simulink model "IEEE_9bus_new_o"  (R2024a)
settings: Solver=ode45  StartTime=0.0  StopTime=10.0  RelTol=1e-3  EnableMultiTasking=on
libraries: spsThreePhaseVIMeasurementLib x21, spsFrequencyPhasorLib x9, spsLoadFlowBusLib x9, spsPower3phInstantaneousLib x9, spsThreePhasePISectionLineLib x6, jailib x3, spsThreePhaseSourceLib x3, spsThreePhaseTransformerTwoWindingsLib x3, sps_lib x1
settings Model: Creator=jp536285  LastModifiedBy=Vaibhav Chaudhary
settings SolverCC: AlgebraicLoopSolver=TrustRegion
settings DataIOCC: LimitDataPoints=on  SaveFormat=Array  ReturnWorkspaceOutputs=off
settings OptimizationCC: LifeSpan=inf
settings DebuggingCC: UnderspecifiedInitializationDetection=Classic  MergeDetectMultiDrivingBlocksExec=none  SolverPrmCheckMsg=warning  StateNameClashWarn=warning  SFUnexpectedBacktrackingDiag=warning  SFNoUnconditionalDefaultTransitionDiag=warning  SFExecutionAtInitializationDiag=none  ArithmeticOperatorsInVariantConditions=warning
settings HardwareCC: ProdBitPerPointer=32  ProdBitPerSizeT=32  ProdBitPerPtrDiffT=32  ProdLargestAtomicFloat=None  ProdIntDivRoundTo=Undefined  ProdEndianess=Unspecified  ProdWordSize=32  ProdHWDeviceType=32-bit Generic
settings ModelReferenceCC: PropagateSignalLabelsOutOfModel=off
settings SFSimCC: SimUseLocalCustomCode=off  CustomCodeUndefinedFunction=UseInterfaceOnly
settings RTWCC: RTWUseLocalCustomCode=off  GPUComputeCapability=3.5
settings CodeAppCC: StateflowObjectComments=on
settings GRTTargetCC: TargetLangStandard=C89/C90 (ANSI)
settings ConfigComp: CovMetricSettings=dw  CovSaveCumulativeToWorkspaceVar=on  CovSaveSingleToWorkspaceVar=on  CovExternalEMLEnable=off
settings SimscapeCC: SimscapeNormalizeSystem=off

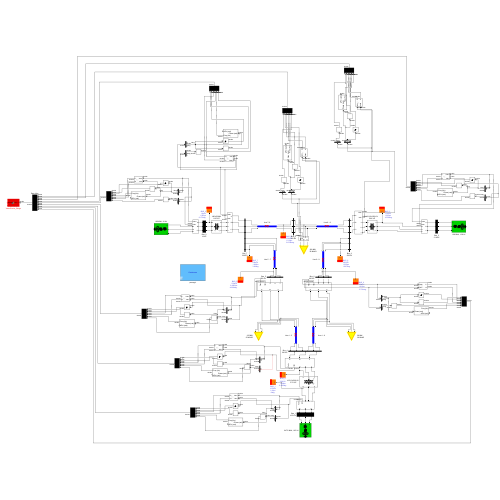
[thumbnail: Simulink's stored preview of the top-level diagram]
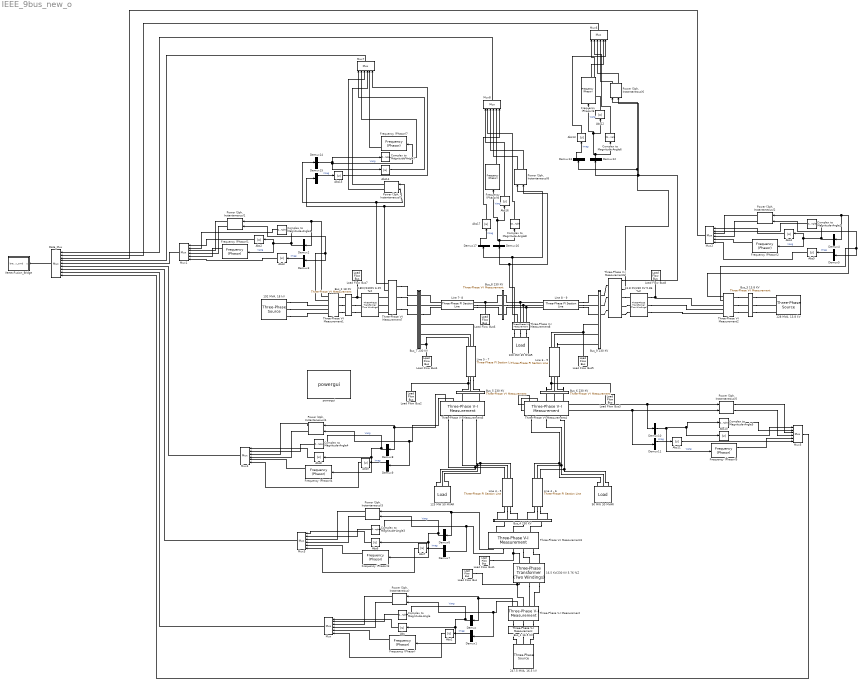
== system IEEE_9bus_new_o ==
  " Line 4 - 6" : spsThreePhasePISectionLineLib/Three-Phase PI Section Line  LConnTagsString=a|b|c  RConnTagsString=A|B|C  Length=100  Frequency=50  Resistances=[ 0.08993 0.224825]  Inductances="[ 1.29e-3  3.22e-3]"  Capacitances=[7.922e-9 4.74e-9]  mask(Three-Phase PI Section Line){}
      mask Display:
      | % This is a new mask on top of the base mask.
      | % Use "View base mask" link below to see the base mask.
      | patch([0.0 0.0 1 1 0.0 0.0 ],[0.4 0.7 0.7 0.4 0.4 0.7],[0 0 1]);
      | patch([0.4 0.4 0.42 0.42],[0.4 0.75 0.75 0.4],[1 0 0]);
      | patch([0.38 0.38 0.57 0.57],[0.7 0.75 0.75 0.7],[1 0 0]);
      | patch([0.53 0.53 0.55 0.55],[0.4 0.75 0.75 0.4],[1 0 0]);
  " Line 6 - 9" : spsThreePhasePISectionLineLib/Three-Phase PI Section Line  LConnTagsString=a|b|c  RConnTagsString=A|B|C  Length=100  Frequency=60  Resistances=[ 0.20631 0.5157]  Inductances="[ 2.38e-3  6.09e-3]"  Capacitances=[17.95e-9 10.55e-9]  mask(Three-Phase PI Section Line){}
      mask Display:
      | % This is a new mask on top of the base mask.
      | % Use "View base mask" link below to see the base mask.
      | patch([0.0 0.0 1 1 0.0 0.0 ],[0.4 0.7 0.7 0.4 0.4 0.7],[0 0 1]);
      | patch([0.4 0.4 0.42 0.42],[0.4 0.75 0.75 0.4],[1 0 0]);
      | patch([0.38 0.38 0.57 0.57],[0.7 0.75 0.75 0.7],[1 0 0]);
      | patch([0.53 0.53 0.55 0.55],[0.4 0.75 0.75 0.4],[1 0 0]);
  100 MW 35 MVAR : jailib/Load  SystemSampleTime=-1  VariantActivationTime=update diagram  AllowFlexibleInterface=on  Latency=0  AutoFrameSizeCalculation=off
      link override Three-Phase Parallel RLC Load: NominalVoltage=230000  ActivePower=100e6  InductivePower=35e6
      settings: SourceProductName=Power Library
  125 MW 50 MVAR : jailib/Load  SystemSampleTime=-1  VariantActivationTime=update diagram  AllowFlexibleInterface=on  Latency=0  AutoFrameSizeCalculation=off
      link override Three-Phase Parallel RLC Load: NominalVoltage=230000  ActivePower=125e6  InductivePower=50e6
      settings: SourceProductName=Power Library
  "128 MVA, 13.8 kV" : spsThreePhaseSourceLib/Three-Phase Source  InternalConnection=Yg  VoltagePhases=off  Voltage=13800  PhaseAngle=0  Voltage_phases=[25e3 25e3 25e3]/sqrt(3)  PhaseAngles_phases=[0 -120 +120]  Frequency=60  NonIdealSource=on  SpecifyImpedance=on  Resistance=0.529  Inductance=0.0140  ShortCircuitLevel=128e6  BaseVoltage=13.8e3  XRratio=100000  BusType=PV  Pref=85000000  Qref=0  Prefabc=[10e3, 10e3, 10e3]  Qrefabc=[0, 0, 0]  Qmin=-inf  Qmax=inf
  13.8 KV/230 KV 5.86 %Z : spsThreePhaseTransformerTwoWindingsLib/Three-Phase Transformer (Two Windings)  Winding1Connection=Yg  Winding2Connection=Yg  CoreType=Three single-phase transformers  SetSaturation=off  Hysteresis=off  DataFile='hysteresis'  SetInitialFlux=off  Measurements=None  UNITS=pu  NominalPower=[ 100e6 , 60 ]  Winding1=[ 13.8e3 , 1e-6 , 0 ]  Winding2=[ 230e3 , 1e-6, 0.0586 ]  Rm=500  Lm=500  L0=0.5  Saturation=[ 0,0 ; 0.0024,1.2 ; 1.0,1.52 ]  InitialFluxes=[ 0.8 , -0.8 , 0.7 ]  BreakLoop=off  DiscreteSolver=Trapezoidal iterative  DataType=off  TransfoNumber=1
  "16.5 KV/230 KV 5.76 %Z     " : spsThreePhaseTransformerTwoWindingsLib/Three-Phase Transformer (Two Windings)  Winding1Connection=Yg  Winding2Connection=Yg  CoreType=Three single-phase transformers  SetSaturation=off  Hysteresis=off  DataFile='hysteresis'  SetInitialFlux=off  Measurements=None  UNITS=pu  NominalPower=[ 100e6 , 60 ]  Winding1=[ 16.5e3 , 1e-6, 0 ]  Winding2=[ 230e3 ,1e-6, 0.0576 ]  Rm=500  Lm=500  L0=0.5  Saturation=[ 0,0 ; 0.0024,1.2 ; 1.0,1.52 ]  InitialFluxes=[ 0.8 , -0.8 , 0.7 ]  BreakLoop=off  DiscreteSolver=Trapezoidal iterative  DataType=off  TransfoNumber=1
  18KV/230KV 6.25 %Z : spsThreePhaseTransformerTwoWindingsLib/Three-Phase Transformer (Two Windings)  Winding1Connection=Yg  Winding2Connection=Yg  CoreType=Three single-phase transformers  SetSaturation=off  Hysteresis=off  DataFile='hysteresis'  SetInitialFlux=off  Measurements=None  UNITS=pu  NominalPower=[ 100e6 , 60 ]  Winding1=[ 18e3 , 1e-6 , 0]  Winding2=[ 230e3 , 1e-6, 0.0625 ]  Rm=500  Lm=500  L0=0.5  Saturation=[ 0,0 ; 0.0024,1.2 ; 1.0,1.52 ]  InitialFluxes=[ 0.8 , -0.8 , 0.7 ]  BreakLoop=off  DiscreteSolver=Trapezoidal iterative  DataType=off  TransfoNumber=1
  "192 MVA, 18 kV" : spsThreePhaseSourceLib/Three-Phase Source  InternalConnection=Yg  VoltagePhases=off  Voltage=18000  PhaseAngle=0  Voltage_phases=[25e3 25e3 25e3]/sqrt(3)  PhaseAngles_phases=[0 -120 +120]  Frequency=60  NonIdealSource=on  SpecifyImpedance=on  Resistance=0.529  Inductance=0.0140  ShortCircuitLevel=192e6  BaseVoltage=18e3  XRratio=100000  BusType=PV  Pref=163000000  Qref=0  Prefabc=[10e3, 10e3, 10e3]  Qrefabc=[0, 0, 0]  Qmin=-inf  Qmax=inf
  "247.5 MVA, 16.5 kV" : spsThreePhaseSourceLib/Three-Phase Source  InternalConnection=Yg  VoltagePhases=off  Voltage=16500  PhaseAngle=0  Voltage_phases=[25e3 25e3 25e3]/sqrt(3)  PhaseAngles_phases=[0 -120 +120]  Frequency=60  NonIdealSource=on  SpecifyImpedance=on  Resistance=0.529  Inductance=0.0140  ShortCircuitLevel=247.5e6  BaseVoltage=16.5e3  XRratio=100000  BusType=swing  Pref=0  Qref=0  Prefabc=[10e3, 10e3, 10e3]  Qrefabc=[0, 0, 0]  Qmin=-Inf  Qmax=Inf
  90 MW 30 MVAR : jailib/Load  SystemSampleTime=-1  VariantActivationTime=update diagram  AllowFlexibleInterface=on  Latency=0  AutoFrameSizeCalculation=off
      link override Three-Phase Parallel RLC Load: NominalVoltage=230000  ActivePower=90e6  InductivePower=30e6
      settings: SourceProductName=Power Library
  Abs{,1..17} (18 alike) : Abs  OutMin=3  OutMax=3  SaturateOnIntegerOverflow=off
  Bus_1 16.5 KV : spsThreePhaseVIMeasurementLib/Three-Phase V-I Measurement  VoltageMeasurement=phase-to-ground  SetLabelV=on  LabelV=Vabc_1  Vpu=on  VpuLL=off  CurrentMeasurement=yes  SetLabelI=on  LabelI=Iabc_1  Ipu=on  Pbase=100e6  Vbase=16.5e3  OutputType=Complex  PhasorSimulation=off  PSBequivalent=0
  Bus_2 18 KV : spsThreePhaseVIMeasurementLib/Three-Phase V-I Measurement  VoltageMeasurement=phase-to-ground  SetLabelV=on  LabelV=Vabc_2  Vpu=on  VpuLL=off  CurrentMeasurement=yes  SetLabelI=on  LabelI=Iabc_2  Ipu=on  Pbase=100e6  Vbase=18e3  OutputType=Complex  PhasorSimulation=off  PSBequivalent=0
  Bus_3 13.8 KV : spsThreePhaseVIMeasurementLib/Three-Phase V-I Measurement  VoltageMeasurement=phase-to-ground  SetLabelV=on  LabelV=Vabc_3  Vpu=on  VpuLL=off  CurrentMeasurement=yes  SetLabelI=on  LabelI=Iabc_3  Ipu=on  Pbase=100e6  Vbase=13.8e3  OutputType=Complex  PhasorSimulation=off  PSBequivalent=0
  Bus_4 230 KV : Subsystem
  Bus_5 230 KV : spsThreePhaseVIMeasurementLib/Three-Phase V-I Measurement  VoltageMeasurement=phase-to-ground  SetLabelV=on  LabelV=Vabc_5  Vpu=on  VpuLL=off  CurrentMeasurement=yes  SetLabelI=on  LabelI=Iabc_5  Ipu=on  Pbase=100e6  Vbase=230e3  OutputType=Complex  PhasorSimulation=off  PSBequivalent=0
  Bus_6 230 KV : spsThreePhaseVIMeasurementLib/Three-Phase V-I Measurement  VoltageMeasurement=phase-to-ground  SetLabelV=on  LabelV=Vabc_6  Vpu=on  VpuLL=off  CurrentMeasurement=yes  SetLabelI=on  LabelI=Iabc_6  Ipu=on  Pbase=100e6  Vbase=230e3  OutputType=Complex  PhasorSimulation=off  PSBequivalent=0
  Bus_7 230 KV : Subsystem
  Bus_8 230 KV : spsThreePhaseVIMeasurementLib/Three-Phase V-I Measurement  VoltageMeasurement=phase-to-ground  SetLabelV=on  LabelV=Vabc_8  Vpu=on  VpuLL=off  CurrentMeasurement=yes  SetLabelI=on  LabelI=Iabc_8  Ipu=on  Pbase=100e6  Vbase=230e3  OutputType=Complex  PhasorSimulation=off  PSBequivalent=0
  Bus_9 230 KV : Subsystem
  Complex to Magnitude-Angle{,1..8} (9 alike) : ComplexToMagnitudeAngle  Output=Angle
  Data_Mux : Mux  Inputs=9
  Demux{,1..17} (18 alike) : Demux  Outputs=3
  Frequency (Phasor){,1..8} (9 alike) : spsFrequencyPhasorLib/Frequency (Phasor)  Fn=60  T=0.1
      settings: LibrarySourceBlock=|
      | sps_lib/Sensors and Measurements/Frequency
      | (Phasor)
  "Line 4 - 5 " : spsThreePhasePISectionLineLib/Three-Phase PI Section Line  LConnTagsString=a|b|c  RConnTagsString=A|B|C  Length=100  Frequency=60  Resistances=[ 0.0529 0.13225]  Inductances="[ 1.192e-3  2.38e-3]"  Capacitances=[8.82e-9 5.188e-9]  mask(Three-Phase PI Section Line){}
      mask Display:
      | % This is a new mask on top of the base mask.
      | % Use "View base mask" link below to see the base mask.
      | patch([0.0 0.0 1 1 0.0 0.0 ],[0.4 0.7 0.7 0.4 0.4 0.7],[0 0 1]);
      | patch([0.4 0.4 0.42 0.42],[0.4 0.75 0.75 0.4],[1 0 0]);
      | patch([0.38 0.38 0.57 0.57],[0.7 0.75 0.75 0.7],[1 0 0]);
      | patch([0.53 0.53 0.55 0.55],[0.4 0.75 0.75 0.4],[1 0 0]);
  "Line 5 - 7 " : spsThreePhasePISectionLineLib/Three-Phase PI Section Line  LConnTagsString=a|b|c  RConnTagsString=A|B|C  Length=100  Frequency=60  Resistances=[ 0.16928 0.4232]  Inductances="[ 2.259e-3  5.64e-3]"  Capacitances=[15.34e-9 9.025e-9]  mask(Three-Phase PI Section Line){}
      mask Display:
      | % This is a new mask on top of the base mask.
      | % Use "View base mask" link below to see the base mask.
      | patch([0.0 0.0 1 1 0.0 0.0 ],[0.4 0.7 0.7 0.4 0.4 0.7],[0 0 1]);
      | patch([0.4 0.4 0.42 0.42],[0.4 0.75 0.75 0.4],[1 0 0]);
      | patch([0.38 0.38 0.57 0.57],[0.7 0.75 0.75 0.7],[1 0 0]);
      | patch([0.53 0.53 0.55 0.55],[0.4 0.75 0.75 0.4],[1 0 0]);
  Line 7- 8 : spsThreePhasePISectionLineLib/Three-Phase PI Section Line  LConnTagsString=a|b|c  RConnTagsString=A|B|C  Length=100  Frequency=60  Resistances=[0.044965 0.11241]  Inductances="[ 1.01e-3  2.02e-3]"  Capacitances=[7.471e-9 4.394e-9]  mask(Three-Phase PI Section Line){}
      mask Display:
      | % This is a new mask on top of the base mask.
      | % Use "View base mask" link below to see the base mask.
      | patch([0.0 0.0 1 1 0.0 0.0 ],[0.4 0.7 0.7 0.4 0.4 0.7],[0 0 1]);
      | patch([0.4 0.4 0.42 0.42],[0.4 0.75 0.75 0.4],[1 0 0]);
      | patch([0.38 0.38 0.57 0.57],[0.7 0.75 0.75 0.7],[1 0 0]);
      | patch([0.53 0.53 0.55 0.55],[0.4 0.75 0.75 0.4],[1 0 0]);
  Line 8 - 9 : spsThreePhasePISectionLineLib/Three-Phase PI Section Line  LConnTagsString=a|b|c  RConnTagsString=A|B|C  Length=100  Frequency=60  Resistances=[ 0.062951 0.15737]  Inductances="[ 1.414e-3  3.53e-3]"  Capacitances=[10.47e-9 6.15e-9]  mask(Three-Phase PI Section Line){}
      mask Display:
      | % This is a new mask on top of the base mask.
      | % Use "View base mask" link below to see the base mask.
      | patch([0.0 0.0 1 1 0.0 0.0 ],[0.4 0.7 0.7 0.4 0.4 0.7],[0 0 1]);
      | patch([0.4 0.4 0.42 0.42],[0.4 0.75 0.75 0.4],[1 0 0]);
      | patch([0.38 0.38 0.57 0.57],[0.7 0.75 0.75 0.7],[1 0 0]);
      | patch([0.53 0.53 0.55 0.55],[0.4 0.75 0.75 0.4],[1 0 0]);
  Load Flow Bus : spsLoadFlowBusLib/Load Flow Bus  LConnTagsString=a  Phases=single  Connectors=on one side  ID=BUS_1  Vbase=16.5e3  Vref=1.04  Vangle=0  VLF=1.04  VLFb=1  VLFc=1  angleLF=0  angleLFb=0  angleLFc=0
      settings: AttributesFormatString=%<ID>\n%<Vbase>V\n%<VLF>pu\n%<angleLF>deg.
  Load Flow Bus1 : spsLoadFlowBusLib/Load Flow Bus  LConnTagsString=a  Phases=single  Connectors=on one side  ID=BUS_4  Vbase=230e3  Vref=1  Vangle=0  VLF=1.026  VLFb=1  VLFc=1  angleLF=-2.226  angleLFb=0  angleLFc=0
      settings: AttributesFormatString=%<ID>\n%<Vbase>V\n%<VLF>pu\n%<angleLF>deg.
  Load Flow Bus2 : spsLoadFlowBusLib/Load Flow Bus  LConnTagsString=a  Phases=single  Connectors=on one side  ID=BUS_5  Vbase=230e3  Vref=1  Vangle=0  VLF=0.9962  VLFb=1  VLFc=1  angleLF=-4.002  angleLFb=0  angleLFc=0
      settings: AttributesFormatString=%<ID>\n%<Vbase>V\n%<VLF>pu\n%<angleLF>deg.
  Load Flow Bus3 : spsLoadFlowBusLib/Load Flow Bus  LConnTagsString=a  Phases=single  Connectors=on one side  ID=BUS_6  Vbase=230e3  Vref=1  Vangle=0  VLF=1.013  VLFb=1  VLFc=1  angleLF=-3.701  angleLFb=0  angleLFc=0
      settings: AttributesFormatString=%<ID>\n%<Vbase>V\n%<VLF>pu\n%<angleLF>deg.
  Load Flow Bus4 : spsLoadFlowBusLib/Load Flow Bus  LConnTagsString=a  Phases=single  Connectors=on one side  ID=BUS_7  Vbase=230e3  Vref=1  Vangle=0  VLF=1.026  VLFb=1  VLFc=1  angleLF=3.62  angleLFb=0  angleLFc=0
      settings: AttributesFormatString=%<ID>\n%<Vbase>V\n%<VLF>pu\n%<angleLF>deg.
  Load Flow Bus5 : spsLoadFlowBusLib/Load Flow Bus  LConnTagsString=a  Phases=single  Connectors=on one side  ID=BUS_9  Vbase=230e3  Vref=1  Vangle=0  VLF=1.032  VLFb=1  VLFc=1  angleLF=1.867  angleLFb=0  angleLFc=0
      settings: AttributesFormatString=%<ID>\n%<Vbase>V\n%<VLF>pu\n%<angleLF>deg.
  Load Flow Bus6 : spsLoadFlowBusLib/Load Flow Bus  LConnTagsString=a  Phases=single  Connectors=on one side  ID=BUS_8  Vbase=230e3  Vref=1  Vangle=0  VLF=1.016  VLFb=1  VLFc=1  angleLF=0.6336  angleLFb=0  angleLFc=0
      settings: AttributesFormatString=%<ID>\n%<Vbase>V\n%<VLF>pu\n%<angleLF>deg.
  Load Flow Bus7 : spsLoadFlowBusLib/Load Flow Bus  LConnTagsString=a  Phases=single  Connectors=on one side  ID=BUS_2  Vbase=18e3  Vref=1.025  Vangle=0  VLF=1.025  VLFb=1  VLFc=1  angleLF=9.173  angleLFb=0  angleLFc=0
      settings: AttributesFormatString=%<ID>\n%<Vbase>V\n%<VLF>pu\n%<angleLF>deg.
  Load Flow Bus8 : spsLoadFlowBusLib/Load Flow Bus  LConnTagsString=a  Phases=single  Connectors=on one side  ID=BUS_3  Vbase=13.8e3  Vref=1.025  Vangle=0  VLF=1.025  VLFb=1  VLFc=1  angleLF=4.558  angleLFb=0  angleLFc=0
      settings: AttributesFormatString=%<ID>\n%<Vbase>V\n%<VLF>pu\n%<angleLF>deg.
  Mux{,1..8} (9 alike) : Mux  Inputs=6
  Power (3ph, Instantaneous){,1..8} (9 alike) : spsPower3phInstantaneousLib/Power (3ph, Instantaneous)
  Three-Phase V-I Measurement{,1..8} (9 alike) : spsThreePhaseVIMeasurementLib/Three-Phase V-I Measurement  VoltageMeasurement=phase-to-ground  SetLabelV=off  LabelV=Vabc  Vpu=on  VpuLL=off  CurrentMeasurement=yes  SetLabelI=off  LabelI=Iabc  Ipu=on  Pbase=100e6  Vbase=500e3  OutputType=Complex  PhasorSimulation=off  PSBequivalent=0
  VertexFusion_Bridge : MATLAB Function  TreatAsAtomicUnit=on
  powergui : sps_lib/powergui  Priority=1  SimulationMode=Continuous  SampleTime=50e-6  frequency=60  Iterations=50  frequencyindice=60  Pbase=10e7  ErrMax=1e-05  UnitsV=kV  UnitsW=MW  buscounter=0  FunctionMessages=off  echomessages=off  EnableUseOfTLC=off  CurrentSourceSwitches=on  DisableSnubberDevices=off  DisableRonSwitches=off  DisableVfSwitches=off  DisplayEquations=off  AutomaticDiscreteSolvers=off  SolverType=Tustin  Interpol=off  ExternalGateDelay=off  methode=off  Ts=0  x0status=blocks  SPID=off  SwTol=0  HookPort=off  NonlinearTolerance=1e-4  nMaxIteration=100  ContinueOnMaxIteration=off  RestoreLinks=warning  ResistiveCurrentMeasurement=off  Frange=[0:2:500]  Ylog=off  Xlog=on  ShowGrid=off  save=off  variable=ZData  structure=0  ZoomFFT=off  StartTime=0.0  cycles=1  DisplayStyle=1  fundamental=60  FreqAxis=off  MaxFrequency=1000  frequencyindicesteady=1  RmsSteady=1  display=off
  wires:
  Three-Phase V-I Measurement/2 -> "Power (3ph, Instantaneous)"/2, Demux1/1
  Demux1/1 -> Abs1/1  "Imag"
  Demux/2 -> Abs/1, Frequency (Phasor)/1, Complex to Magnitude-Angle/1  "Vang"
  Three-Phase V-I Measurement/1 -> "Power (3ph, Instantaneous)"/1, Demux/1
  Abs/1 -> Mux/1
  Complex to Magnitude-Angle/1 -> Mux/2
  "Power (3ph, Instantaneous)"/1 -> Mux/3
  "Power (3ph, Instantaneous)"/2 -> Mux/4
  Frequency (Phasor)/1 -> Mux/5
  Abs1/1 -> Mux/6
  Demux2/2 -> Abs2/1, Frequency (Phasor)1/1, Complex to Magnitude-Angle1/1  "Vang"
  Frequency (Phasor)1/1 -> Mux1/5
  Abs2/1 -> Mux1/1
  Complex to Magnitude-Angle1/1 -> Mux1/2
  Abs3/1 -> Mux1/6
  Demux3/1 -> Abs3/1  "Imag"
  "Power (3ph, Instantaneous)1"/2 -> Mux1/4
  "Power (3ph, Instantaneous)1"/1 -> Mux1/3
  Three-Phase V-I Measurement1/2 -> "Power (3ph, Instantaneous)1"/2, Demux3/1
  Three-Phase V-I Measurement1/1 -> Demux2/1, "Power (3ph, Instantaneous)1"/1
  Three-Phase V-I Measurement2/2 -> "Power (3ph, Instantaneous)2"/2, Demux5/1
  Three-Phase V-I Measurement2/1 -> Demux4/1, "Power (3ph, Instantaneous)2"/1
  "Power (3ph, Instantaneous)2"/1 -> Mux2/3
  "Power (3ph, Instantaneous)2"/2 -> Mux2/4
  Abs5/1 -> Mux2/6
  Abs4/1 -> Mux2/1
  Complex to Magnitude-Angle2/1 -> Mux2/2
  Frequency (Phasor)2/1 -> Mux2/5
  Demux5/1 -> Abs5/1  "Imag"
  Demux4/2 -> Abs4/1, Frequency (Phasor)2/1, Complex to Magnitude-Angle2/1  "Vang"
  Demux6/2 -> Abs6/1, Frequency (Phasor)3/1, Complex to Magnitude-Angle3/1  "Vang"
  Frequency (Phasor)3/1 -> Mux3/5
  Abs6/1 -> Mux3/1
  Complex to Magnitude-Angle3/1 -> Mux3/2
  Abs7/1 -> Mux3/6
  Demux7/1 -> Abs7/1  "Imag"
  "Power (3ph, Instantaneous)3"/2 -> Mux3/4
  "Power (3ph, Instantaneous)3"/1 -> Mux3/3
  Three-Phase V-I Measurement3/2 -> "Power (3ph, Instantaneous)3"/2
  Three-Phase V-I Measurement3/1 -> "Power (3ph, Instantaneous)3"/1, Demux6/1
  Demux8/2 -> Abs8/1, Frequency (Phasor)4/1, Complex to Magnitude-Angle4/1  "Vang"
  Frequency (Phasor)4/1 -> Mux4/5
  Abs8/1 -> Mux4/1
  Complex to Magnitude-Angle4/1 -> Mux4/2
  Abs9/1 -> Mux4/6
  Demux9/1 -> Abs9/1  "Imag"
  "Power (3ph, Instantaneous)4"/2 -> Mux4/4
  "Power (3ph, Instantaneous)4"/1 -> Mux4/3
  Three-Phase V-I Measurement5/2 -> "Power (3ph, Instantaneous)4"/2, Demux9/1
  Three-Phase V-I Measurement5/1 -> "Power (3ph, Instantaneous)4"/1, Demux8/1
  Demux10/2 -> Abs10/1, Complex to Magnitude-Angle5/1, Frequency (Phasor)5/1  "Vang"
  Frequency (Phasor)5/1 -> Mux5/5
  Abs10/1 -> Mux5/1
  Complex to Magnitude-Angle5/1 -> Mux5/2
  Abs11/1 -> Mux5/6
  Demux11/1 -> Abs11/1  "Imag"
  "Power (3ph, Instantaneous)5"/2 -> Mux5/4
  "Power (3ph, Instantaneous)5"/1 -> Mux5/3
  Three-Phase V-I Measurement4/2 -> Demux11/1, "Power (3ph, Instantaneous)5"/2
  Three-Phase V-I Measurement4/1 -> Demux10/1, "Power (3ph, Instantaneous)5"/1
  Demux13/1 -> Abs13/1  "Imag"
  Demux12/2 -> Abs12/1, Frequency (Phasor)6/1, Complex to Magnitude-Angle6/1  "Vang"
  "Power (3ph, Instantaneous)6"/1 -> Mux6/3
  Abs12/1 -> Mux6/1
  "Power (3ph, Instantaneous)6"/2 -> Mux6/4
  Complex to Magnitude-Angle6/1 -> Mux6/2
  Frequency (Phasor)6/1 -> Mux6/5
  Three-Phase V-I Measurement6/2 -> "Power (3ph, Instantaneous)6"/2, Demux13/1
  Three-Phase V-I Measurement6/1 -> Demux12/1, "Power (3ph, Instantaneous)6"/1
  Abs13/1 -> Mux6/6
  Three-Phase V-I Measurement7/2 -> "Power (3ph, Instantaneous)7"/2, Demux15/1
  Three-Phase V-I Measurement7/1 -> Demux14/1, "Power (3ph, Instantaneous)7"/1
  "Power (3ph, Instantaneous)7"/1 -> Mux7/3
  Demux15/1 -> Abs15/1  "Imag"
  Abs14/1 -> Mux7/1
  Complex to Magnitude-Angle7/1 -> Mux7/2
  Demux14/2 -> Complex to Magnitude-Angle7/1, Abs14/1, Frequency (Phasor)7/1  "Vang"
  Abs15/1 -> Mux7/6
  Frequency (Phasor)7/1 -> Mux7/5
  "Power (3ph, Instantaneous)7"/2 -> Mux7/4
  Three-Phase V-I Measurement8/1 -> "Power (3ph, Instantaneous)8"/1, Demux16/1
  Abs17/1 -> Mux8/6
  "Power (3ph, Instantaneous)8"/2 -> Mux8/4
  Abs16/1 -> Mux8/1
  Complex to Magnitude-Angle8/1 -> Mux8/2
  Frequency (Phasor)8/1 -> Mux8/5
  "Power (3ph, Instantaneous)8"/1 -> Mux8/3
  Demux17/1 -> Abs17/1  "Imag"
  Demux16/2 -> Abs16/1, Frequency (Phasor)8/1, Complex to Magnitude-Angle8/1  "Vang"
  Three-Phase V-I Measurement8/2 -> "Power (3ph, Instantaneous)8"/2, Demux17/1
  Mux1/1 -> Data_Mux/5
  Mux4/1 -> Data_Mux/6
  Mux3/1 -> Data_Mux/7
  Mux/1 -> Data_Mux/8
  Mux5/1 -> Data_Mux/9
  Mux7/1 -> Data_Mux/4
  Mux8/1 -> Data_Mux/1
  Mux6/1 -> Data_Mux/2
  Mux2/1 -> Data_Mux/3
  Data_Mux/1 -> VertexFusion_Bridge/1(u)
  connections:
  Load Flow Bus7/LConn1 -- Bus_2 18 KV/RConn1 -- 18KV/230KV 6.25 %Z/LConn1
  13.8 KV/230 KV 5.86 %Z/LConn1 -- Three-Phase V-I Measurement2/RConn1 -- Load Flow Bus8/LConn1
  Bus_1 16.5 KV/RConn1 -- "247.5 MVA, 16.5 kV"/RConn1
  Bus_1 16.5 KV/RConn2 -- "247.5 MVA, 16.5 kV"/RConn2
  Bus_1 16.5 KV/RConn3 -- "247.5 MVA, 16.5 kV"/RConn3
  Load Flow Bus/LConn1 -- Three-Phase V-I Measurement/RConn1 -- "16.5 KV/230 KV 5.76 %Z     "/LConn1
  Load Flow Bus1/LConn1 -- Three-Phase V-I Measurement3/RConn1 -- "16.5 KV/230 KV 5.76 %Z     "/RConn1
  Line 8 - 9/LConn1 -- Three-Phase V-I Measurement8/RConn1 -- Bus_8 230 KV/LConn1
  Bus_8 230 KV/LConn2 -- Line 8 - 9/LConn2 -- Three-Phase V-I Measurement8/RConn2
  Line 8 - 9/LConn3 -- Three-Phase V-I Measurement8/RConn3 -- Bus_8 230 KV/LConn3
  125 MW 50 MVAR/LConn1 -- "Line 4 - 5 "/LConn1 -- Three-Phase V-I Measurement5/LConn1
  125 MW 50 MVAR/LConn2 -- "Line 4 - 5 "/LConn2 -- Three-Phase V-I Measurement5/LConn2
  125 MW 50 MVAR/LConn3 -- Three-Phase V-I Measurement5/LConn3 -- "Line 4 - 5 "/LConn3
  " Line 4 - 6"/LConn1 -- Three-Phase V-I Measurement4/LConn1 -- 90 MW 30 MVAR/LConn1
  " Line 4 - 6"/LConn2 -- Three-Phase V-I Measurement4/LConn2 -- 90 MW 30 MVAR/LConn2
  " Line 4 - 6"/LConn3 -- Three-Phase V-I Measurement4/LConn3 -- 90 MW 30 MVAR/LConn3
  Line 7- 8/LConn1 -- Bus_7 230 KV/RConn1
  Line 7- 8/LConn2 -- Bus_7 230 KV/RConn2
  Bus_7 230 KV/RConn3 -- Line 7- 8/LConn3
  Bus_8 230 KV/RConn1 -- Load Flow Bus6/LConn1 -- Line 7- 8/RConn1
  Line 7- 8/RConn2 -- Bus_8 230 KV/RConn2
  Line 7- 8/RConn3 -- Bus_8 230 KV/RConn3
  Line 8 - 9/RConn2 -- Bus_9 230 KV/LConn2
  Line 8 - 9/RConn1 -- Bus_9 230 KV/LConn1
  Line 8 - 9/RConn3 -- Bus_9 230 KV/LConn3
  "Line 5 - 7 "/RConn1 -- Bus_5 230 KV/LConn1 -- Load Flow Bus2/LConn1
  "Line 5 - 7 "/RConn2 -- Bus_5 230 KV/LConn2
  "Line 5 - 7 "/RConn3 -- Bus_5 230 KV/LConn3
  "Line 5 - 7 "/LConn1 -- Load Flow Bus4/LConn1 -- Bus_7 230 KV/RConn6
  "Line 5 - 7 "/LConn2 -- Bus_7 230 KV/RConn5
  "Line 5 - 7 "/LConn3 -- Bus_7 230 KV/RConn4
  " Line 6 - 9"/RConn1 -- Load Flow Bus5/LConn1 -- Bus_9 230 KV/LConn4
  Bus_9 230 KV/LConn5 -- " Line 6 - 9"/RConn2
  Bus_6 230 KV/LConn1 -- Load Flow Bus3/LConn1 -- " Line 6 - 9"/LConn1
  Bus_6 230 KV/LConn2 -- " Line 6 - 9"/LConn2
  Bus_6 230 KV/LConn3 -- " Line 6 - 9"/LConn3
  " Line 6 - 9"/RConn3 -- Bus_9 230 KV/LConn6
  "Line 4 - 5 "/RConn2 -- Bus_4 230 KV/RConn2
  "Line 4 - 5 "/RConn1 -- Bus_4 230 KV/RConn1
  "Line 4 - 5 "/RConn3 -- Bus_4 230 KV/RConn3
  " Line 4 - 6"/RConn2 -- Bus_4 230 KV/RConn5
  " Line 4 - 6"/RConn1 -- Bus_4 230 KV/RConn4
  " Line 4 - 6"/RConn3 -- Bus_4 230 KV/RConn6
  Bus_3 13.8 KV/RConn1 -- "128 MVA, 13.8 kV"/RConn1
  Bus_3 13.8 KV/RConn2 -- "128 MVA, 13.8 kV"/RConn2
  Bus_3 13.8 KV/RConn3 -- "128 MVA, 13.8 kV"/RConn3
  Three-Phase V-I Measurement/LConn3 -- Bus_1 16.5 KV/LConn3
  Three-Phase V-I Measurement/LConn2 -- Bus_1 16.5 KV/LConn2
  Three-Phase V-I Measurement/LConn1 -- Bus_1 16.5 KV/LConn1
  "16.5 KV/230 KV 5.76 %Z     "/LConn3 -- Three-Phase V-I Measurement/RConn3
  "16.5 KV/230 KV 5.76 %Z     "/LConn2 -- Three-Phase V-I Measurement/RConn2
  Bus_2 18 KV/RConn2 -- 18KV/230KV 6.25 %Z/LConn2
  Bus_2 18 KV/RConn3 -- 18KV/230KV 6.25 %Z/LConn3
  Three-Phase V-I Measurement1/LConn2 -- Bus_2 18 KV/LConn2
  Three-Phase V-I Measurement1/LConn1 -- Bus_2 18 KV/LConn1
  Three-Phase V-I Measurement1/LConn3 -- Bus_2 18 KV/LConn3
  "192 MVA, 18 kV"/RConn1 -- Three-Phase V-I Measurement1/RConn1
  "192 MVA, 18 kV"/RConn2 -- Three-Phase V-I Measurement1/RConn2
  "192 MVA, 18 kV"/RConn3 -- Three-Phase V-I Measurement1/RConn3
  Three-Phase V-I Measurement2/LConn3 -- Bus_3 13.8 KV/LConn3
  Three-Phase V-I Measurement2/LConn2 -- Bus_3 13.8 KV/LConn2
  Three-Phase V-I Measurement2/LConn1 -- Bus_3 13.8 KV/LConn1
  13.8 KV/230 KV 5.86 %Z/LConn2 -- Three-Phase V-I Measurement2/RConn2
  13.8 KV/230 KV 5.86 %Z/LConn3 -- Three-Phase V-I Measurement2/RConn3
  Three-Phase V-I Measurement3/RConn3 -- "16.5 KV/230 KV 5.76 %Z     "/RConn3
  Three-Phase V-I Measurement3/RConn2 -- "16.5 KV/230 KV 5.76 %Z     "/RConn2
  Bus_4 230 KV/LConn3 -- Three-Phase V-I Measurement3/LConn3
  Bus_4 230 KV/LConn2 -- Three-Phase V-I Measurement3/LConn2
  Bus_4 230 KV/LConn1 -- Three-Phase V-I Measurement3/LConn1
  Three-Phase V-I Measurement4/RConn3 -- Bus_6 230 KV/RConn3
  Three-Phase V-I Measurement4/RConn2 -- Bus_6 230 KV/RConn2
  Three-Phase V-I Measurement4/RConn1 -- Bus_6 230 KV/RConn1
  Three-Phase V-I Measurement5/RConn3 -- Bus_5 230 KV/RConn3
  Three-Phase V-I Measurement5/RConn1 -- Bus_5 230 KV/RConn1
  Three-Phase V-I Measurement6/RConn3 -- 13.8 KV/230 KV 5.86 %Z/RConn3
  Three-Phase V-I Measurement6/RConn2 -- 13.8 KV/230 KV 5.86 %Z/RConn2
  Three-Phase V-I Measurement6/RConn1 -- 13.8 KV/230 KV 5.86 %Z/RConn1
  Bus_9 230 KV/RConn1 -- Three-Phase V-I Measurement6/LConn1
  Bus_9 230 KV/RConn2 -- Three-Phase V-I Measurement6/LConn2
  Bus_9 230 KV/RConn3 -- Three-Phase V-I Measurement6/LConn3
  Three-Phase V-I Measurement7/RConn1 -- 18KV/230KV 6.25 %Z/RConn1
  Three-Phase V-I Measurement7/RConn3 -- 18KV/230KV 6.25 %Z/RConn3
  Three-Phase V-I Measurement7/RConn2 -- 18KV/230KV 6.25 %Z/RConn2
  Three-Phase V-I Measurement7/LConn3 -- Bus_7 230 KV/LConn3
  Three-Phase V-I Measurement7/LConn2 -- Bus_7 230 KV/LConn2
  Three-Phase V-I Measurement7/LConn1 -- Bus_7 230 KV/LConn1
  Three-Phase V-I Measurement8/LConn3 -- 100 MW 35 MVAR/LConn3
  Three-Phase V-I Measurement8/LConn2 -- 100 MW 35 MVAR/LConn2
  Three-Phase V-I Measurement8/LConn1 -- 100 MW 35 MVAR/LConn1

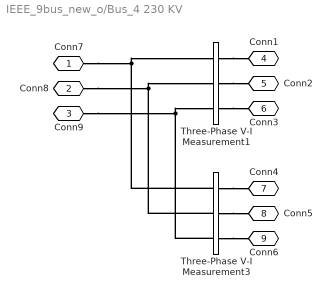
== system IEEE_9bus_new_o/Bus_4 230 KV ==
  Three-Phase V-I Measurement1 : spsThreePhaseVIMeasurementLib/Three-Phase V-I Measurement  VoltageMeasurement=phase-to-ground  SetLabelV=on  LabelV=Vabc_45  Vpu=on  VpuLL=off  CurrentMeasurement=yes  SetLabelI=on  LabelI=Iabc_45  Ipu=on  Pbase=100e6  Vbase=230e3  OutputType=Complex  PhasorSimulation=off  PSBequivalent=0
  Three-Phase V-I Measurement3 : spsThreePhaseVIMeasurementLib/Three-Phase V-I Measurement  VoltageMeasurement=phase-to-ground  SetLabelV=on  LabelV=Vabc_46  Vpu=on  VpuLL=off  CurrentMeasurement=yes  SetLabelI=on  LabelI=Iabc_46  Ipu=on  Pbase=100e6  Vbase=230e3  OutputType=Complex  PhasorSimulation=off  PSBequivalent=0
  Conn7 : PMIOPort  Side=Left
  Conn8 : PMIOPort  Port=2  Side=Left
  Conn9 : PMIOPort  Port=3  Side=Left
  Conn1 : PMIOPort  Port=4  Side=Right
  Conn2 : PMIOPort  Port=5  Side=Right
  Conn3 : PMIOPort  Port=6  Side=Right
  Conn4 : PMIOPort  Port=7  Side=Right
  Conn5 : PMIOPort  Port=8  Side=Right
  Conn6 : PMIOPort  Port=9  Side=Right
  connections:
  Three-Phase V-I Measurement3/LConn3 -- Conn9/RConn1 -- Three-Phase V-I Measurement1/LConn3
  Three-Phase V-I Measurement3/LConn2 -- Conn8/RConn1 -- Three-Phase V-I Measurement1/LConn2
  Three-Phase V-I Measurement3/LConn1 -- Conn7/RConn1 -- Three-Phase V-I Measurement1/LConn1
  Three-Phase V-I Measurement3/RConn3 -- Conn6/RConn1
  Three-Phase V-I Measurement1/RConn3 -- Conn3/RConn1
  Three-Phase V-I Measurement1/RConn1 -- Conn1/RConn1
  Three-Phase V-I Measurement1/RConn2 -- Conn2/RConn1
  Three-Phase V-I Measurement3/RConn1 -- Conn4/RConn1
  Three-Phase V-I Measurement3/RConn2 -- Conn5/RConn1

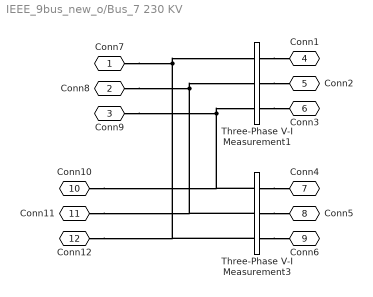
== system IEEE_9bus_new_o/Bus_7 230 KV ==
  Three-Phase V-I Measurement1 : spsThreePhaseVIMeasurementLib/Three-Phase V-I Measurement  VoltageMeasurement=phase-to-ground  SetLabelV=on  LabelV=Vabc_7  Vpu=on  VpuLL=off  CurrentMeasurement=yes  SetLabelI=on  LabelI=Iabc_7  Ipu=on  Pbase=100e6  Vbase=230e3  OutputType=Complex  PhasorSimulation=off  PSBequivalent=0
  Three-Phase V-I Measurement3 : spsThreePhaseVIMeasurementLib/Three-Phase V-I Measurement  VoltageMeasurement=phase-to-ground  SetLabelV=on  LabelV=Vab  Vpu=on  VpuLL=off  CurrentMeasurement=yes  SetLabelI=on  LabelI=Iab  Ipu=on  Pbase=100e6  Vbase=230e3  OutputType=Complex  PhasorSimulation=off  PSBequivalent=0
  Conn7 : PMIOPort  Side=Left
  Conn8 : PMIOPort  Port=2  Side=Left
  Conn9 : PMIOPort  Port=3  Side=Left
  Conn1 : PMIOPort  Port=4  Side=Right
  Conn2 : PMIOPort  Port=5  Side=Right
  Conn3 : PMIOPort  Port=6  Side=Right
  Conn4 : PMIOPort  Port=7  Side=Right
  Conn5 : PMIOPort  Port=8  Side=Right
  Conn6 : PMIOPort  Port=9  Side=Right
  Conn10 : PMIOPort  Port=10  Side=Left
  Conn11 : PMIOPort  Port=11  Side=Left
  Conn12 : PMIOPort  Port=12  Side=Left
  connections:
  Three-Phase V-I Measurement3/RConn2 -- Conn5/RConn1
  Three-Phase V-I Measurement3/RConn1 -- Conn4/RConn1
  Three-Phase V-I Measurement1/RConn2 -- Conn2/RConn1
  Three-Phase V-I Measurement1/RConn1 -- Conn1/RConn1
  Three-Phase V-I Measurement1/RConn3 -- Conn3/RConn1
  Three-Phase V-I Measurement3/RConn3 -- Conn6/RConn1
  Conn7/RConn1 -- Three-Phase V-I Measurement3/LConn3 -- Conn12/RConn1 -- Three-Phase V-I Measurement1/LConn1
  Conn8/RConn1 -- Three-Phase V-I Measurement3/LConn2 -- Conn11/RConn1 -- Three-Phase V-I Measurement1/LConn2
  Conn9/RConn1 -- Conn10/RConn1 -- Three-Phase V-I Measurement3/LConn1 -- Three-Phase V-I Measurement1/LConn3

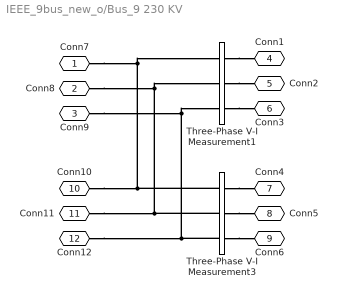
== system IEEE_9bus_new_o/Bus_9 230 KV ==
  Three-Phase V-I Measurement1 : spsThreePhaseVIMeasurementLib/Three-Phase V-I Measurement  VoltageMeasurement=phase-to-ground  SetLabelV=on  LabelV=Vabc_9  Vpu=on  VpuLL=off  CurrentMeasurement=yes  SetLabelI=on  LabelI=Iabc_9  Ipu=on  Pbase=100e6  Vbase=230e3  OutputType=Complex  PhasorSimulation=off  PSBequivalent=0
  Three-Phase V-I Measurement3 : spsThreePhaseVIMeasurementLib/Three-Phase V-I Measurement  VoltageMeasurement=phase-to-ground  SetLabelV=on  LabelV=Vabc  Vpu=on  VpuLL=off  CurrentMeasurement=yes  SetLabelI=on  LabelI=Iabc  Ipu=on  Pbase=100e6  Vbase=230e3  OutputType=Complex  PhasorSimulation=off  PSBequivalent=0
  Conn7 : PMIOPort  Side=Left
  Conn8 : PMIOPort  Port=2  Side=Left
  Conn9 : PMIOPort  Port=3  Side=Left
  Conn1 : PMIOPort  Port=4  Side=Right
  Conn2 : PMIOPort  Port=5  Side=Right
  Conn3 : PMIOPort  Port=6  Side=Right
  Conn4 : PMIOPort  Port=7  Side=Right
  Conn5 : PMIOPort  Port=8  Side=Right
  Conn6 : PMIOPort  Port=9  Side=Right
  Conn10 : PMIOPort  Port=10  Side=Left
  Conn11 : PMIOPort  Port=11  Side=Left
  Conn12 : PMIOPort  Port=12  Side=Left
  connections:
  Conn12/RConn1 -- Three-Phase V-I Measurement3/LConn3 -- Conn9/RConn1 -- Three-Phase V-I Measurement1/LConn3
  Conn11/RConn1 -- Three-Phase V-I Measurement3/LConn2 -- Conn8/RConn1 -- Three-Phase V-I Measurement1/LConn2
  Conn10/RConn1 -- Three-Phase V-I Measurement3/LConn1 -- Conn7/RConn1 -- Three-Phase V-I Measurement1/LConn1
  Three-Phase V-I Measurement3/RConn3 -- Conn6/RConn1
  Three-Phase V-I Measurement1/RConn3 -- Conn3/RConn1
  Three-Phase V-I Measurement1/RConn1 -- Conn1/RConn1
  Three-Phase V-I Measurement1/RConn2 -- Conn2/RConn1
  Three-Phase V-I Measurement3/RConn1 -- Conn4/RConn1
  Three-Phase V-I Measurement3/RConn2 -- Conn5/RConn1

== matlab function IEEE_9bus_new_o/VertexFusion_Bridge ==
  data: breaker_cmd output double size=[1 1]; u input size=[54 1]
function breaker_cmd = tcp_sync_logic(u)
% Vertex Fusion TCP Sync Logic (Simulink Coder Optimized)
% This function sends 54 IEEE 9-bus features to Python AI Hub.

% 1. Declare extrinsic and persistent variables at the TOP-LEVEL
coder.extrinsic('tcpclient', 'write', 'read', 'isempty', 'strcmp');
persistent tcp_client;

% 2. Pre-initialize output as a double scalar (Crucial for Coder)
breaker_cmd = 1.0; 

% 3. Handle 54-feature vector safety check
if length(u) ~= 54
    return;
end

% 4. Extrinsic logic for Simulation/Interpretation
if coder.target('MATLAB')
    % Lazy connect
    if isempty(tcp_client)
        try
            tcp_client = tcpclient('127.0.0.1', 5000, 'Timeout', 0.1);
        catch
            % If server is unreachable, we keep breaker_cmd = 1
            return;
        end
    end
    
    % Communication logic
    if ~isempty(tcp_client)
        % Send features
        write(tcp_client, u, 'double');
        
        % Check for mitigation command (4 bytes: 'TRIP' or 'NORM')
        if tcp_client.NumBytesAvailable >= 4
            % Read exactly 4 chars
            cmd_raw = read(tcp_client, 4, 'char');
            
            % Use strcmp (extrinsic) for safe comparison
            if strcmp(cmd_raw, 'TRIP')
                breaker_cmd = 0.0;
            else
                breaker_cmd = 1.0;
            end
        end
    end
end

end
